simulink model "Peak_Shave_Model"  (R2020a)
settings: Solver=FixedStepAuto  StartTime=0.0  StopTime=24  FixedStep=0.001  RelTol=1e-3
undefined symbols (not defined in the file): auxPower, BESSCapacity, deliveryPrice1, deliveryPrice2, deliveryPrice3, deliveryPrice4, efficiency, EVCapacity, midPeakChargeSetting, midPeakDischargeSetting, MidPeakHours1, MidPeakHours2, MidPeakHoursOverflow1, MidPeakHoursOverflow2, MidPeakHoursOverflowStatus, MidPeakPrice, MURBOverload, offPeakChargeSetting, offPeakDischargeSetting, OffPeakHours1, OffPeakHours2, OffPeakHoursOverflow1, OffPeakHoursOverflow2, OffPeakHoursOverflowStatus, OffPeakPrice, onPeakChargeSetting, onPeakDischargeSetting, OnPeakHours1, OnPeakHours2, OnPeakHours3, OnPeakHours4, OnPeakHoursOverflow1, OnPeakHoursOverflow2, OnPeakHoursOverflow3, OnPeakHoursOverflow4, OnPeakHoursOverflowStatus1, OnPeakHoursOverflowStatus2, OnPeakPrice, ratedPower, ratedPowerNEG, tier1Price, tier2Price, tierRateKW
libraries: simulink x21
settings Model: Creator=jeffm  LastModifiedBy=jeffm
settings DataIOCC: ExternalInput=ts  LoadExternalInput=on

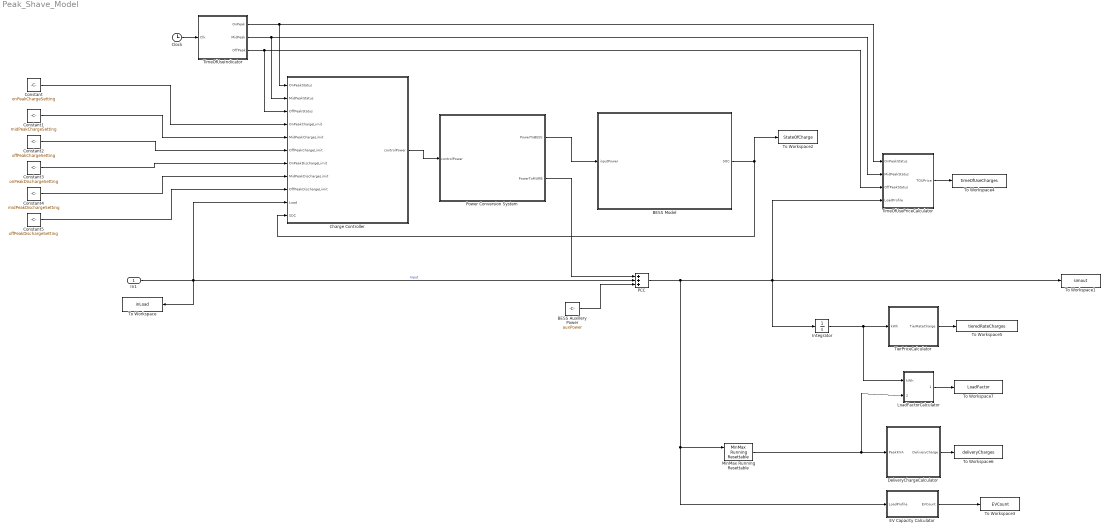
== system Peak_Shave_Model ==
  In1 : Inport
  BESS Auxillery Power : Constant  Value=auxPower  VectorParams1D=off
  BESS Model : Subsystem
  Charge Controller : Subsystem
  Clock : Clock
  Constant : Constant  Value=onPeakChargeSetting
      settings: AttributesFormatString=%<Value>
  Constant1 : Constant  Value=midPeakChargeSetting
      settings: AttributesFormatString=%<Value>
  Constant2 : Constant  Value=offPeakChargeSetting
      settings: AttributesFormatString=%<Value>
  Constant3 : Constant  Value=onPeakDischargeSetting
      settings: AttributesFormatString=%<Value>
  Constant4 : Constant  Value=midPeakDischargeSetting
      settings: AttributesFormatString=%<Value>
  Constant5 : Constant  Value=offPeakDischargeSetting
      settings: AttributesFormatString=%<Value>
  DeliveryChargeCalculator : Subsystem
  EV Capacity Calculator : Subsystem
  Integrator : Integrator
  LoadFactorCalculator : Subsystem
  MinMax Running Resettable : simulink/Math Operations/MinMax Running Resettable  Function=max  vinit=0.0
  PCC : Sum  Inputs=+++
  Power Conversion System : Subsystem
  TierPriceCalculator : Subsystem
  TimeOfUseIndicator : Subsystem
  TimeOfUsePriceCalculator : Subsystem
  To Workspace : ToWorkspace  VariableName=inLoad  SaveFormat=Timeseries  SampleTime=-1
  To Workspace1 : ToWorkspace  VariableName=simout  SaveFormat=Timeseries  SampleTime=-1
  To Workspace2 : ToWorkspace  VariableName=StateOfCharge  SaveFormat=Timeseries  SampleTime=-1
  To Workspace3 : ToWorkspace  VariableName=EVCount  SaveFormat=Timeseries  SampleTime=-1
  To Workspace4 : ToWorkspace  VariableName=timeOfUseCharges  SaveFormat=Timeseries  SampleTime=-1
      settings: MaxDataPoints=1
  To Workspace5 : ToWorkspace  VariableName=tieredRateCharges  SaveFormat=Timeseries  SampleTime=-1
      settings: MaxDataPoints=1
  To Workspace6 : ToWorkspace  VariableName=deliveryCharges  SaveFormat=Timeseries  SampleTime=-1
      settings: MaxDataPoints=1
  To Workspace7 : ToWorkspace  VariableName=LoadFactor  SaveFormat=Timeseries  SampleTime=-1
      settings: MaxDataPoints=1
  wires:
  In1/1 -> Charge Controller/10(Load), To Workspace/1, PCC/2  "Input"
  Power Conversion System/2(PowerToMURB) -> PCC/1
  BESS Auxillery Power/1 -> PCC/3
  PCC/1 -> TimeOfUsePriceCalculator/4(LoadProfile), Integrator/1, To Workspace1/1, EV Capacity Calculator/1(LoadProfile), MinMax Running Resettable/1
  Charge Controller/1(controlPower) -> Power Conversion System/1(controlPower)
  Power Conversion System/1(PowerToBESS) -> BESS Model/1(inputPower)
  BESS Model/1(SOC) -> Charge Controller/11(SOC), To Workspace2/1
  Clock/1 -> TimeOfUseIndicator/1(Clk)
  Constant/1 -> Charge Controller/4(OnPeakChargeLimit)
  Constant1/1 -> Charge Controller/5(MidPeakChargeLimit)
  Constant2/1 -> Charge Controller/6(OffPeakChargeLimit)
  Constant3/1 -> Charge Controller/7(OnPeakDischargeLimit)
  Constant4/1 -> Charge Controller/8(MidPeakDischargeLimit)
  Constant5/1 -> Charge Controller/9(OffPeakDischargeLimit)
  TimeOfUseIndicator/1(OnPeak) -> TimeOfUsePriceCalculator/1(OnPeakStatus), Charge Controller/1(OnPeakStatus)
  TimeOfUseIndicator/2(MidPeak) -> Charge Controller/2(MidPeakStatus), TimeOfUsePriceCalculator/2(MidPeakStatus)
  TimeOfUseIndicator/3(OffPeak) -> Charge Controller/3(OffPeakStatus), TimeOfUsePriceCalculator/3(OffPeakStatus)
  EV Capacity Calculator/1(EVCount) -> To Workspace3/1
  TimeOfUsePriceCalculator/1(TOUPrice) -> To Workspace4/1
  Integrator/1 -> TierPriceCalculator/1(kWh), LoadFactorCalculator/1(kWh)
  TierPriceCalculator/1(TierRateCharge) -> To Workspace5/1
  MinMax Running Resettable/1 -> LoadFactorCalculator/2(peakKVA), DeliveryChargeCalculator/1(PeakKVA)
  DeliveryChargeCalculator/1(DeliveryCharge) -> To Workspace6/1
  LoadFactorCalculator/1(LoadFactor) -> To Workspace7/1

== system Peak_Shave_Model/BESS Model ==
  inputPower : Inport
  BESS Capacity : Saturate  UpperLimit=BESSCapacity  LowerLimit=0
  Energy Conversion : Integrator
  Gain : Gain  Gain=100*(1/BESSCapacity)
  SOC : Outport
  wires:
  Energy Conversion/1 -> BESS Capacity/1
  BESS Capacity/1 -> Gain/1
  Gain/1 -> SOC/1  "SOC"
  inputPower/1 -> Energy Conversion/1

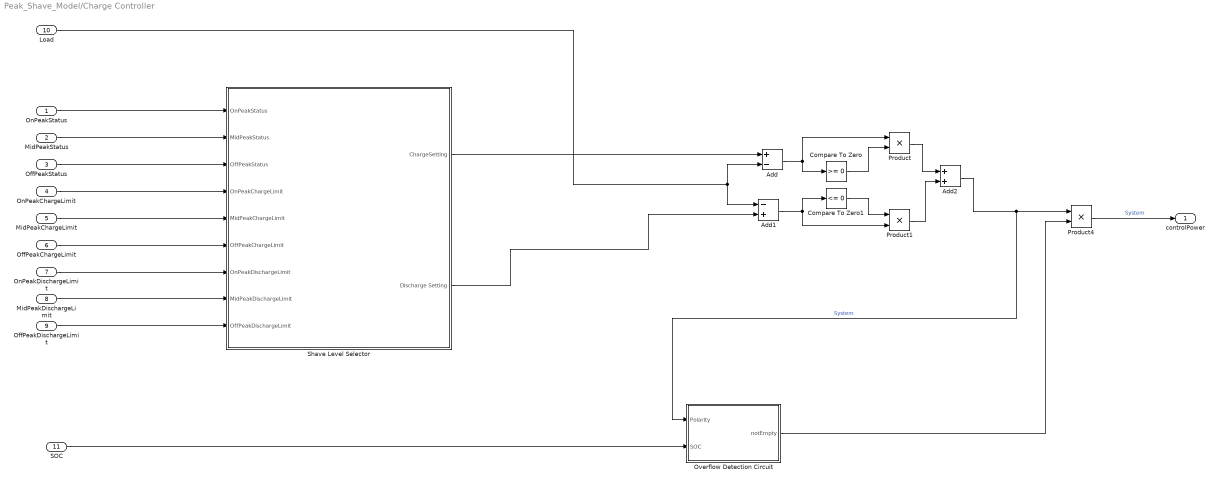
== system Peak_Shave_Model/Charge Controller ==
  OnPeakStatus : Inport
  MidPeakStatus : Inport  Port=2
  OffPeakStatus : Inport  Port=3
  OnPeakChargeLimit : Inport  Port=4
  MidPeakChargeLimit : Inport  Port=5
  OffPeakChargeLimit : Inport  Port=6
  OnPeakDischargeLimit : Inport  Port=7
  MidPeakDischargeLimit : Inport  Port=8
  OffPeakDischargeLimit : Inport  Port=9
  Load : Inport  Port=10
  SOC : Inport  Port=11
  Add : Sum  Inputs=+-
  Add1 : Sum  Inputs=-+
  Add2 : Sum
  Compare To Zero : simulink/Logic and Bit Operations/Compare To Zero  relop=>=  OutDataTypeStr=boolean
  Compare To Zero1 : simulink/Logic and Bit Operations/Compare To Zero  relop=<=  OutDataTypeStr=boolean
  Overflow Detection Circuit : Subsystem
  Product : Product
  Product1 : Product
  Product4 : Product
  Shave Level Selector : Subsystem
  controlPower : Outport
  wires:
  Compare To Zero/1 -> Product/2
  Add/1 -> Product/1, Compare To Zero/1
  Add1/1 -> Compare To Zero1/1, Product1/2
  Compare To Zero1/1 -> Product1/1
  Product/1 -> Add2/1
  Load/1 -> Add/2, Add1/1
  Add2/1 -> Overflow Detection Circuit/1(Polarity), Product4/1  "System"
  Product1/1 -> Add2/2
  Product4/1 -> controlPower/1  "System"
  OnPeakChargeLimit/1 -> Shave Level Selector/4(OnPeakChargeLimit)
  MidPeakChargeLimit/1 -> Shave Level Selector/5(MidPeakChargeLimit)
  OffPeakChargeLimit/1 -> Shave Level Selector/6(OffPeakChargeLimit)
  OnPeakDischargeLimit/1 -> Shave Level Selector/7(OnPeakDischargeLimit)
  MidPeakDischargeLimit/1 -> Shave Level Selector/8(MidPeakDischargeLimit)
  OffPeakDischargeLimit/1 -> Shave Level Selector/9(OffPeakDischargeLimit)
  Shave Level Selector/1(ChargeSetting) -> Add/1
  Shave Level Selector/2(Discharge Setting) -> Add1/2
  SOC/1 -> Overflow Detection Circuit/2(SOC)
  Overflow Detection Circuit/1(notEmpty) -> Product4/2
  OnPeakStatus/1 -> Shave Level Selector/1(OnPeakStatus)
  MidPeakStatus/1 -> Shave Level Selector/2(MidPeakStatus)
  OffPeakStatus/1 -> Shave Level Selector/3(OffPeakStatus)

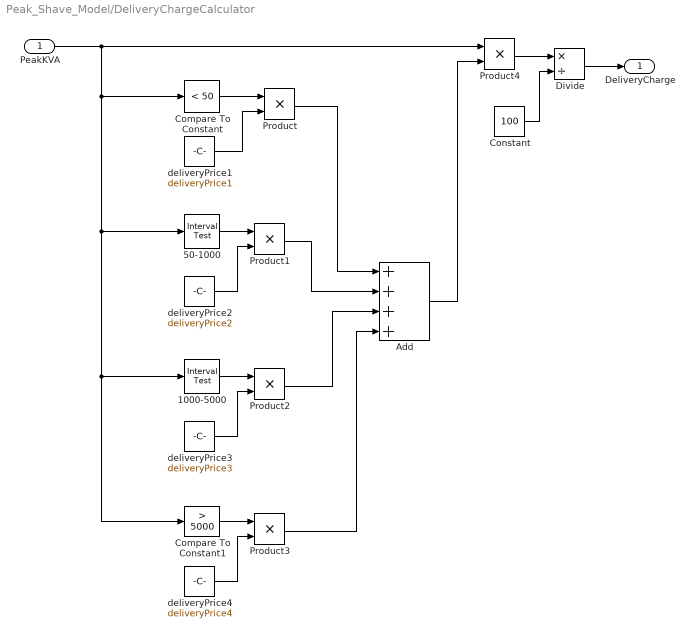
== system Peak_Shave_Model/DeliveryChargeCalculator ==
  PeakKVA : Inport
  1000-5000 : simulink/Logic and Bit Operations/Interval Test  IntervalClosedRight=off  uplimit=5000  IntervalClosedLeft=on  lowlimit=1000  OutDataTypeStr=boolean
  50-1000 : simulink/Logic and Bit Operations/Interval Test  IntervalClosedRight=off  uplimit=1000  IntervalClosedLeft=on  lowlimit=50  OutDataTypeStr=boolean
  Add : Sum  Inputs=++++
  Compare To Constant : simulink/Logic and Bit Operations/Compare To Constant  relop=<  const=50  OutDataTypeStr=boolean
  Compare To Constant1 : simulink/Logic and Bit Operations/Compare To Constant  relop=>  const=5000  OutDataTypeStr=boolean
  Constant : Constant  Value=100
  Divide : Product  Inputs=*/
  Product{,1..4} (5 alike) : Product
  deliveryPrice1 : Constant  Value=deliveryPrice1
  deliveryPrice2 : Constant  Value=deliveryPrice2
  deliveryPrice3 : Constant  Value=deliveryPrice3
  deliveryPrice4 : Constant  Value=deliveryPrice4
  DeliveryCharge : Outport
  wires:
  PeakKVA/1 -> Compare To Constant1/1, 1000-5000/1, 50-1000/1, Compare To Constant/1, Product4/1
  deliveryPrice1/1 -> Product/2
  Compare To Constant/1 -> Product/1
  50-1000/1 -> Product1/1
  deliveryPrice2/1 -> Product1/2
  deliveryPrice3/1 -> Product2/2
  1000-5000/1 -> Product2/1
  deliveryPrice4/1 -> Product3/2
  Compare To Constant1/1 -> Product3/1
  Product/1 -> Add/1
  Product1/1 -> Add/2
  Product2/1 -> Add/3
  Product3/1 -> Add/4
  Add/1 -> Product4/2
  Constant/1 -> Divide/2
  Product4/1 -> Divide/1
  Divide/1 -> DeliveryCharge/1

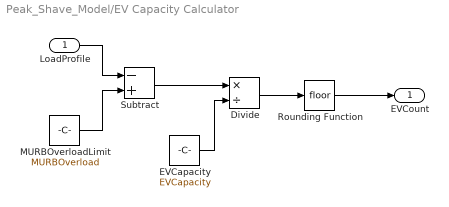
== system Peak_Shave_Model/EV Capacity Calculator ==
  LoadProfile : Inport
  Divide : Product  Inputs=*/
  EVCapacity : Constant  Value=EVCapacity
  MURBOverloadLimit : Constant  Value=MURBOverload
  Rounding Function : Rounding
  Subtract : Sum  Inputs=-+
  EVCount : Outport
  wires:
  Subtract/1 -> Divide/1
  EVCapacity/1 -> Divide/2
  Rounding Function/1 -> EVCount/1
  LoadProfile/1 -> Subtract/1
  Divide/1 -> Rounding Function/1
  MURBOverloadLimit/1 -> Subtract/2

== system Peak_Shave_Model/LoadFactorCalculator ==
  kWh : Inport
  peakKVA : Inport  Port=2
  Constant6 : Constant  Value=24
  Divide : Product  Inputs=*/
  Product : Product
  LoadFactor : Outport
  wires:
  Constant6/1 -> Product/2
  Product/1 -> Divide/2
  Divide/1 -> LoadFactor/1
  kWh/1 -> Divide/1
  peakKVA/1 -> Product/1

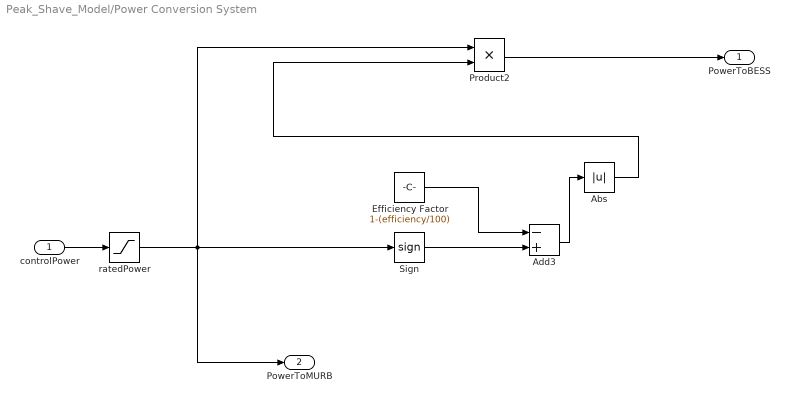
== system Peak_Shave_Model/Power Conversion System ==
  controlPower : Inport
  Abs : Abs
  Add3 : Sum  Inputs=-+
  Efficiency Factor : Constant  Value=1-(efficiency/100)
  Product2 : Product
  Sign : Signum
  ratedPower : Saturate  UpperLimit=ratedPower  LowerLimit=ratedPowerNEG
  PowerToBESS : Outport
  PowerToMURB : Outport  Port=2
  wires:
  ratedPower/1 -> PowerToMURB/1, Sign/1, Product2/1
  Abs/1 -> Product2/2
  controlPower/1 -> ratedPower/1
  Sign/1 -> Add3/2
  Add3/1 -> Abs/1
  Product2/1 -> PowerToBESS/1
  Efficiency Factor/1 -> Add3/1

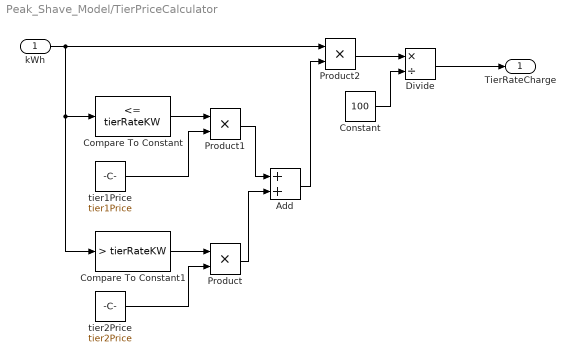
== system Peak_Shave_Model/TierPriceCalculator ==
  kWh : Inport
  Add : Sum
  Compare To Constant : simulink/Logic and Bit Operations/Compare To Constant  relop=<=  const=tierRateKW  OutDataTypeStr=boolean
  Compare To Constant1 : simulink/Logic and Bit Operations/Compare To Constant  relop=>  const=tierRateKW  OutDataTypeStr=boolean
  Constant : Constant  Value=100
  Divide : Product  Inputs=*/
  Product : Product
  Product1 : Product
  Product2 : Product
  tier1Price : Constant  Value=tier1Price
  tier2Price : Constant  Value=tier2Price
  TierRateCharge : Outport
  wires:
  kWh/1 -> Compare To Constant1/1, Compare To Constant/1, Product2/1
  tier2Price/1 -> Product/2
  Compare To Constant1/1 -> Product/1
  tier1Price/1 -> Product1/2
  Compare To Constant/1 -> Product1/1
  Product1/1 -> Add/1
  Product/1 -> Add/2
  Add/1 -> Product2/2
  Constant/1 -> Divide/2
  Product2/1 -> Divide/1
  Divide/1 -> TierRateCharge/1

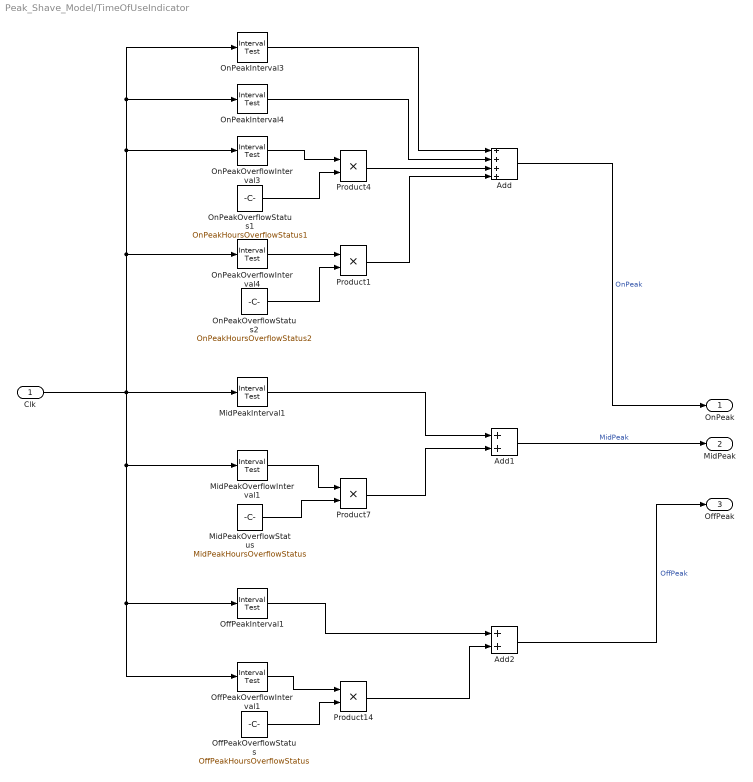
== system Peak_Shave_Model/TimeOfUseIndicator ==
  Clk : Inport
  Add : Sum  Inputs=++++
  Add1 : Sum
  Add2 : Sum
  MidPeakInterval1 : simulink/Logic and Bit Operations/Interval Test  IntervalClosedRight=off  uplimit=MidPeakHours2  IntervalClosedLeft=on  lowlimit=MidPeakHours1  OutDataTypeStr=boolean
  MidPeakOverflowInterval1 : simulink/Logic and Bit Operations/Interval Test  IntervalClosedRight=off  uplimit=MidPeakHoursOverflow2  IntervalClosedLeft=on  lowlimit=MidPeakHoursOverflow1  OutDataTypeStr=boolean
  MidPeakOverflowStatus : Constant  Value=MidPeakHoursOverflowStatus
  OffPeakInterval1 : simulink/Logic and Bit Operations/Interval Test  IntervalClosedRight=off  uplimit=OffPeakHours2  IntervalClosedLeft=on  lowlimit=OffPeakHours1  OutDataTypeStr=boolean
  OffPeakOverflowInterval1 : simulink/Logic and Bit Operations/Interval Test  IntervalClosedRight=off  uplimit=OffPeakHoursOverflow2  IntervalClosedLeft=on  lowlimit=OffPeakHoursOverflow1  OutDataTypeStr=boolean
  OffPeakOverflowStatus : Constant  Value=OffPeakHoursOverflowStatus
  OnPeakInterval3 : simulink/Logic and Bit Operations/Interval Test  IntervalClosedRight=off  uplimit=OnPeakHours2  IntervalClosedLeft=on  lowlimit=OnPeakHours1  OutDataTypeStr=boolean
  OnPeakInterval4 : simulink/Logic and Bit Operations/Interval Test  IntervalClosedRight=off  uplimit=OnPeakHours4  IntervalClosedLeft=on  lowlimit=OnPeakHours3  OutDataTypeStr=boolean
  OnPeakOverflowInterval3 : simulink/Logic and Bit Operations/Interval Test  IntervalClosedRight=off  uplimit=OnPeakHoursOverflow2  IntervalClosedLeft=on  lowlimit=OnPeakHoursOverflow1  OutDataTypeStr=boolean
  OnPeakOverflowInterval4 : simulink/Logic and Bit Operations/Interval Test  IntervalClosedRight=off  uplimit=OnPeakHoursOverflow4  IntervalClosedLeft=on  lowlimit=OnPeakHoursOverflow3  OutDataTypeStr=boolean
  OnPeakOverflowStatus1 : Constant  Value=OnPeakHoursOverflowStatus1
  OnPeakOverflowStatus2 : Constant  Value=OnPeakHoursOverflowStatus2
  Product{1,4,7,14} (4 alike) : Product
  OnPeak : Outport
  MidPeak : Outport  Port=2
  OffPeak : Outport  Port=3
  wires:
  Product4/1 -> Add/3
  Product7/1 -> Add1/2
  Product1/1 -> Add/4
  Product14/1 -> Add2/2
  Add/1 -> OnPeak/1  "OnPeak"
  Add2/1 -> OffPeak/1  "OffPeak"
  Add1/1 -> MidPeak/1  "MidPeak"
  OnPeakInterval3/1 -> Add/1
  OnPeakInterval4/1 -> Add/2
  OnPeakOverflowInterval3/1 -> Product4/1
  OnPeakOverflowInterval4/1 -> Product1/1
  MidPeakInterval1/1 -> Add1/1
  MidPeakOverflowInterval1/1 -> Product7/1
  OffPeakInterval1/1 -> Add2/1
  OffPeakOverflowInterval1/1 -> Product14/1
  OnPeakOverflowStatus1/1 -> Product4/2
  OnPeakOverflowStatus2/1 -> Product1/2
  MidPeakOverflowStatus/1 -> Product7/2
  OffPeakOverflowStatus/1 -> Product14/2
  Clk/1 -> MidPeakOverflowInterval1/1, OffPeakInterval1/1, OffPeakOverflowInterval1/1, MidPeakInterval1/1, OnPeakOverflowInterval4/1, OnPeakOverflowInterval3/1, OnPeakInterval4/1, OnPeakInterval3/1

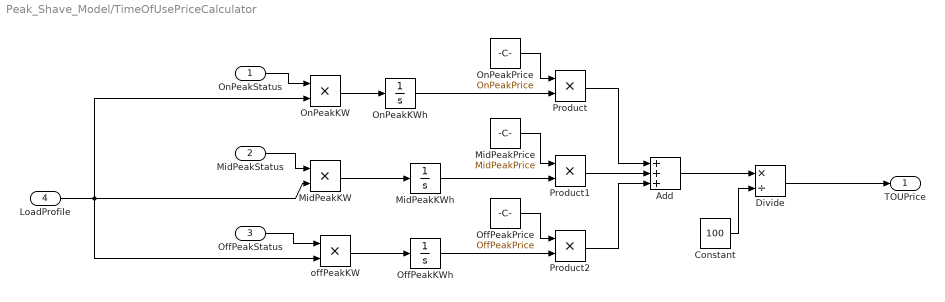
== system Peak_Shave_Model/TimeOfUsePriceCalculator ==
  OnPeakStatus : Inport
  MidPeakStatus : Inport  Port=2
  OffPeakStatus : Inport  Port=3
  LoadProfile : Inport  Port=4
  Add : Sum  Inputs=+++
  Constant : Constant  Value=100
  Divide : Product  Inputs=*/
  MidPeakKW : Product
  MidPeakKWh : Integrator
  MidPeakPrice : Constant  Value=MidPeakPrice
  OffPeakKWh : Integrator
  OffPeakPrice : Constant  Value=OffPeakPrice
  OnPeakKW : Product
  OnPeakKWh : Integrator
  OnPeakPrice : Constant  Value=OnPeakPrice
  Product : Product
  Product1 : Product
  Product2 : Product
  offPeakKW : Product
  TOUPrice : Outport
  wires:
  offPeakKW/1 -> OffPeakKWh/1
  LoadProfile/1 -> offPeakKW/2, MidPeakKW/2, OnPeakKW/2
  MidPeakStatus/1 -> MidPeakKW/1
  OnPeakKW/1 -> OnPeakKWh/1
  MidPeakKW/1 -> MidPeakKWh/1
  OnPeakStatus/1 -> OnPeakKW/1
  OffPeakStatus/1 -> offPeakKW/1
  OnPeakPrice/1 -> Product/1
  OnPeakKWh/1 -> Product/2
  MidPeakKWh/1 -> Product1/2
  MidPeakPrice/1 -> Product1/1
  OffPeakPrice/1 -> Product2/1
  OffPeakKWh/1 -> Product2/2
  Product/1 -> Add/1
  Product1/1 -> Add/2
  Product2/1 -> Add/3
  Constant/1 -> Divide/2
  Add/1 -> Divide/1
  Divide/1 -> TOUPrice/1

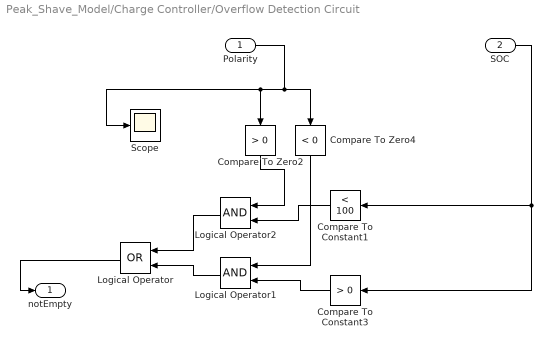
== system Peak_Shave_Model/Charge Controller/Overflow Detection Circuit ==
  Polarity : Inport
  SOC : Inport  Port=2
  Compare To Constant1 : simulink/Logic and Bit Operations/Compare To Constant  relop=<  const=100  OutDataTypeStr=boolean
  Compare To Constant3 : simulink/Logic and Bit Operations/Compare To Constant  relop=>  const=0  OutDataTypeStr=boolean
  Compare To Zero2 : simulink/Logic and Bit Operations/Compare To Zero  relop=>  OutDataTypeStr=boolean
  Compare To Zero4 : simulink/Logic and Bit Operations/Compare To Zero  relop=<  OutDataTypeStr=boolean
  Logical Operator : Logic  Operator=OR  AllPortsSameDT=off  OutDataTypeStr=boolean
  Logical Operator1 : Logic  AllPortsSameDT=off  OutDataTypeStr=boolean
  Logical Operator2 : Logic  AllPortsSameDT=off  OutDataTypeStr=boolean
  Scope : Scope
  notEmpty : Outport
  wires:
  SOC/1 -> Compare To Constant3/1, Compare To Constant1/1
  Logical Operator1/1 -> Logical Operator/2
  Compare To Zero4/1 -> Logical Operator1/1
  Compare To Zero2/1 -> Logical Operator2/1
  Logical Operator2/1 -> Logical Operator/1
  Polarity/1 -> Scope/1, Compare To Zero2/1, Compare To Zero4/1
  Logical Operator/1 -> notEmpty/1
  Compare To Constant3/1 -> Logical Operator1/2
  Compare To Constant1/1 -> Logical Operator2/2

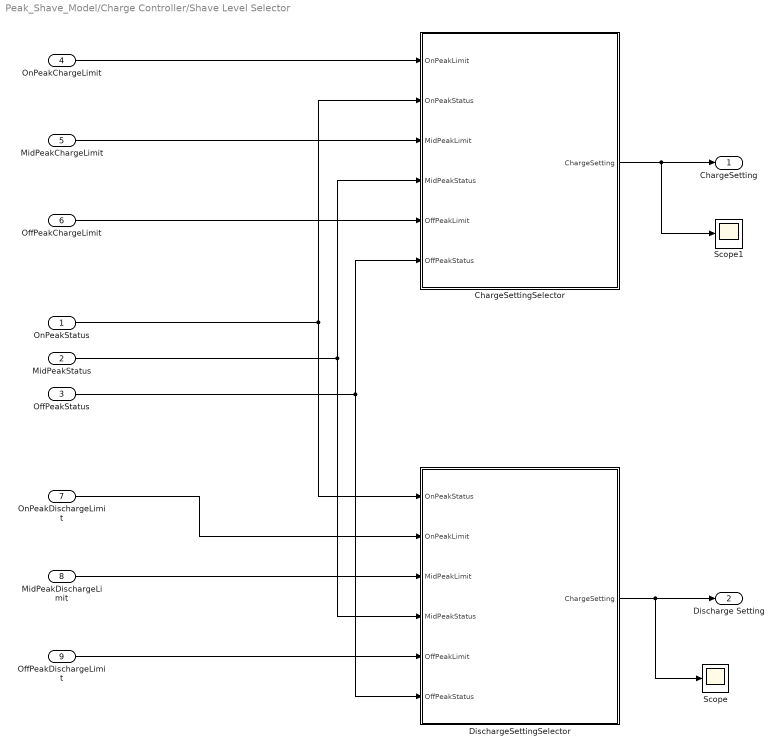
== system Peak_Shave_Model/Charge Controller/Shave Level Selector ==
  OnPeakStatus : Inport
  MidPeakStatus : Inport  Port=2
  OffPeakStatus : Inport  Port=3
  OnPeakChargeLimit : Inport  Port=4
  MidPeakChargeLimit : Inport  Port=5
  OffPeakChargeLimit : Inport  Port=6
  OnPeakDischargeLimit : Inport  Port=7
  MidPeakDischargeLimit : Inport  Port=8
  OffPeakDischargeLimit : Inport  Port=9
  ChargeSettingSelector : Subsystem
  DischargeSettingSelector : Subsystem
  Scope : Scope
  Scope1 : Scope
  ChargeSetting : Outport
  Discharge Setting : Outport  Port=2
  wires:
  MidPeakChargeLimit/1 -> ChargeSettingSelector/3(MidPeakLimit)
  OnPeakChargeLimit/1 -> ChargeSettingSelector/1(OnPeakLimit)
  OffPeakChargeLimit/1 -> ChargeSettingSelector/5(OffPeakLimit)
  DischargeSettingSelector/1(ChargeSetting) -> Scope/1, Discharge Setting/1
  ChargeSettingSelector/1(ChargeSetting) -> Scope1/1, ChargeSetting/1
  OnPeakDischargeLimit/1 -> DischargeSettingSelector/2(OnPeakLimit)
  MidPeakDischargeLimit/1 -> DischargeSettingSelector/3(MidPeakLimit)
  OffPeakDischargeLimit/1 -> DischargeSettingSelector/5(OffPeakLimit)
  OnPeakStatus/1 -> DischargeSettingSelector/1(OnPeakStatus), ChargeSettingSelector/2(OnPeakStatus)
  MidPeakStatus/1 -> DischargeSettingSelector/4(MidPeakStatus), ChargeSettingSelector/4(MidPeakStatus)
  OffPeakStatus/1 -> ChargeSettingSelector/6(OffPeakStatus), DischargeSettingSelector/6(OffPeakStatus)

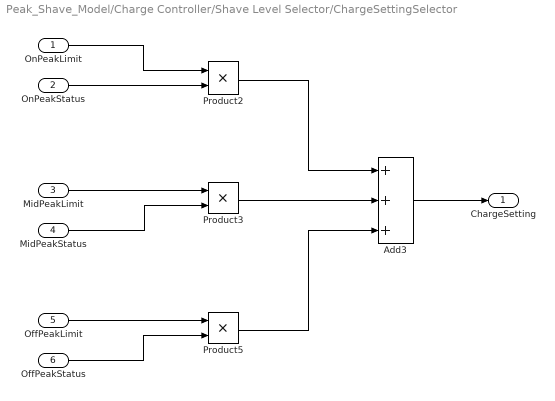
== system Peak_Shave_Model/Charge Controller/Shave Level Selector/ChargeSettingSelector ==
  OnPeakLimit : Inport
  OnPeakStatus : Inport  Port=2
  MidPeakLimit : Inport  Port=3
  MidPeakStatus : Inport  Port=4
  OffPeakLimit : Inport  Port=5
  OffPeakStatus : Inport  Port=6
  Add3 : Sum  Inputs=+++
  Product2 : Product
  Product3 : Product
  Product5 : Product
  ChargeSetting : Outport
  wires:
  MidPeakLimit/1 -> Product3/1
  OffPeakLimit/1 -> Product5/1
  OnPeakLimit/1 -> Product2/1
  Product2/1 -> Add3/1
  Add3/1 -> ChargeSetting/1
  Product3/1 -> Add3/2
  Product5/1 -> Add3/3
  OnPeakStatus/1 -> Product2/2
  MidPeakStatus/1 -> Product3/2
  OffPeakStatus/1 -> Product5/2

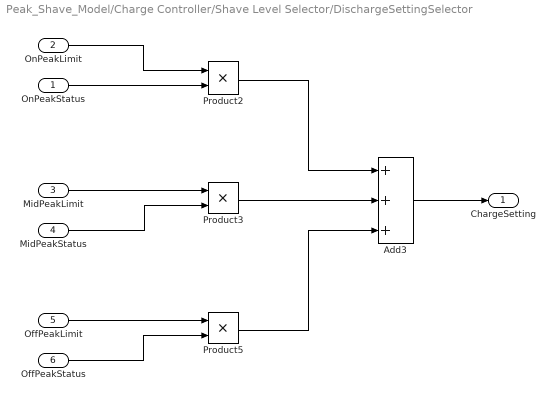
== system Peak_Shave_Model/Charge Controller/Shave Level Selector/DischargeSettingSelector ==
  OnPeakStatus : Inport
  OnPeakLimit : Inport  Port=2
  MidPeakLimit : Inport  Port=3
  MidPeakStatus : Inport  Port=4
  OffPeakLimit : Inport  Port=5
  OffPeakStatus : Inport  Port=6
  Add3 : Sum  Inputs=+++
  Product2 : Product
  Product3 : Product
  Product5 : Product
  ChargeSetting : Outport
  wires:
  MidPeakLimit/1 -> Product3/1
  OffPeakLimit/1 -> Product5/1
  OnPeakLimit/1 -> Product2/1
  Product2/1 -> Add3/1
  Add3/1 -> ChargeSetting/1
  Product3/1 -> Add3/2
  Product5/1 -> Add3/3
  OnPeakStatus/1 -> Product2/2
  MidPeakStatus/1 -> Product3/2
  OffPeakStatus/1 -> Product5/2
